simulink model "PID_example_incorrect"  (R2012b)
settings: Solver=ode1  StartTime=0.0  StopTime=80  FixedStep=0.01  RelTol=1e-3
StopFcn:
  | plot(time,[Input simout simout1]);legend('Input','Anti Windup','Incorrect');grid;
  | title('What happens with incorrect implementation')
  | xlabel('Time (sec)');ylabel('Magnitude')
  | shg
undefined symbols (not defined in the file): sigbuilder_block
libraries: simulink x2
settings Model: Creator=JYOGANAN  LastModifiedBy=JYOGANAN

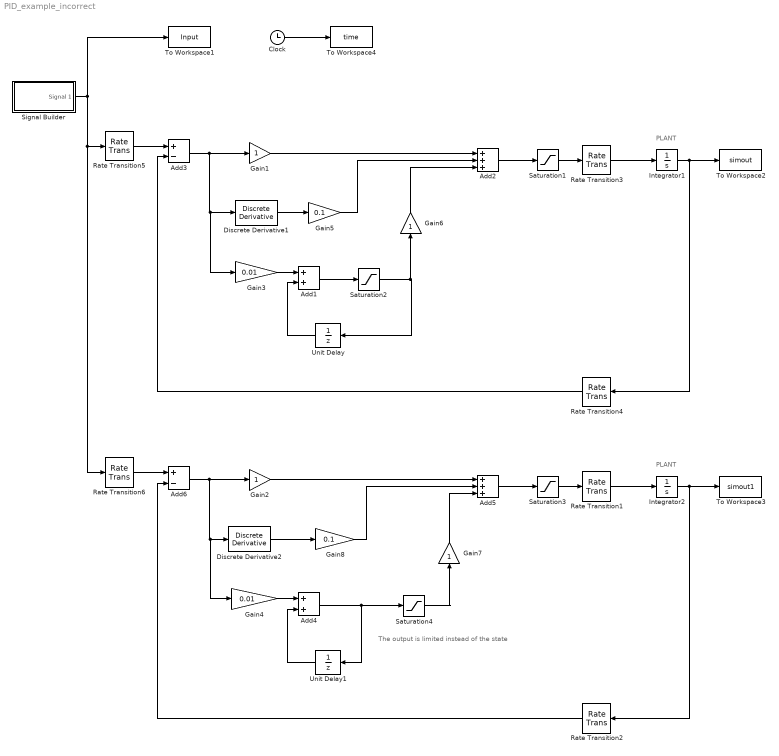
== system PID_example_incorrect ==
  note: The output is limited instead of the state
  note: PLANT
  note: PLANT
  Add1 : Sum
  Add2 : Sum  Inputs=+++
  Add3 : Sum  Inputs=+-
  Add4 : Sum
  Add5 : Sum  Inputs=+++
  Add6 : Sum  Inputs=+-
  Clock : Clock
  Discrete Derivative1 : simulink/Discrete/Discrete Derivative  gainval=1.0  ICPrevScaledInput=0.0  InputProcessing=Inherited  OutMin=[]  OutMax=[]  OutDataType=fixdt(1, 16)  OutScaling=2^-10  DoSatur=off
  Discrete Derivative2 : simulink/Discrete/Discrete Derivative  gainval=1.0  ICPrevScaledInput=0.0  InputProcessing=Inherited  OutMin=[]  OutMax=[]  OutDataType=fixdt(1, 16)  OutScaling=2^-10  DoSatur=off
  Gain{1..2,6..7} (4 alike) : Gain
  Gain3 : Gain  Gain=0.01
  Gain4 : Gain  Gain=0.01
  Gain5 : Gain  Gain=0.1
  Gain8 : Gain  Gain=0.1
  Integrator1 : Integrator
  Integrator2 : Integrator
  Rate Transition1 : RateTransition
  Rate Transition{2,4..6} (4 alike) : RateTransition  OutPortSampleTime=0.01
  Rate Transition3 : RateTransition
  Saturation1 : Saturate  UpperLimit=1  LowerLimit=-1
  Saturation2 : Saturate
  Saturation3 : Saturate  UpperLimit=1  LowerLimit=-1
  Saturation4 : Saturate
  Signal Builder : Subsystem  Tag=STV Subsys  LoadFcn=sigbuilder_block('load');  StartFcn=sigbuilder_block('start');  StopFcn=sigbuilder_block('stop');  ClipboardFcn=sigbuilder_block('clipboard');  mask(Sigbuilder block){}
      mask help: Simulink:masks:SigbuilderBlock_MD
      mask init:
      | if ~strcmp(get_param(bdroot(gcbh),'SimulationStatus'),'stopped') tuvar = sigbuilder_block('maskInit'); end
      settings: CopyFcn=sigbuilder_block('copy');  DeleteFcn=sigbuilder_block('delete');  ModelCloseFcn=sigbuilder_block('modelClose');  PreSaveFcn=sigbuilder_block('preSave');  PauseFcn=sigbuilder_block('pause');  ContinueFcn=sigbuilder_block('continue');  NameChangeFcn=sigbuilder_block('namechange');  OpenFcn=sigbuilder_block('open',[406.5 147 550.5 399.75 ]);  CloseFcn=sigbuilder_block('close');
      mask Display: plot(0, 0, 100, 100,[2, 2, 32, 32, 2], [68, 8, 8, 68, 68],[32, 2], [38, 38], [32, 19, 2],[53, 60, 44], [32, 17, 17, 2],[16, 16, 31, 31]);txt = getActiveGroup(gcbh);text(2, 100, txt,'verticalAlignment', 'top');
  To Workspace1 : ToWorkspace  VariableName=Input  SampleTime=-1
  To Workspace2 : ToWorkspace  VariableName=simout  SampleTime=-1
  To Workspace3 : ToWorkspace  VariableName=simout1  SampleTime=-1
  To Workspace4 : ToWorkspace  VariableName=time  SampleTime=-1
  Unit Delay : UnitDelay  SampleTime=-1
  Unit Delay1 : UnitDelay  SampleTime=-1
  wires:
  Rate Transition3/1 -> Integrator1/1
  Gain1/1 -> Add2/1
  Rate Transition4/1 -> Add3/2
  Integrator1/1 -> To Workspace2/1, Rate Transition4/1
  Rate Transition5/1 -> Add3/1
  Discrete Derivative1/1 -> Gain5/1
  Saturation1/1 -> Rate Transition3/1
  Add2/1 -> Saturation1/1
  Add3/1 -> Gain3/1, Discrete Derivative1/1, Gain1/1
  Signal Builder/1(Signal 1) -> To Workspace1/1, Rate Transition5/1, Rate Transition6/1
  Clock/1 -> To Workspace4/1
  Add1/1 -> Saturation2/1
  Gain3/1 -> Add1/1
  Unit Delay/1 -> Add1/2
  Saturation2/1 -> Unit Delay/1, Gain6/1
  Rate Transition1/1 -> Integrator2/1
  Gain2/1 -> Add5/1
  Rate Transition2/1 -> Add6/2
  Integrator2/1 -> To Workspace3/1, Rate Transition2/1
  Rate Transition6/1 -> Add6/1
  Discrete Derivative2/1 -> Gain8/1
  Saturation3/1 -> Rate Transition1/1
  Add5/1 -> Saturation3/1
  Add6/1 -> Gain4/1, Discrete Derivative2/1, Gain2/1
  Gain4/1 -> Add4/1
  Unit Delay1/1 -> Add4/2
  Add4/1 -> Saturation4/1, Unit Delay1/1
  Saturation4/1 -> Gain7/1
  Gain5/1 -> Add2/2
  Gain6/1 -> Add2/3
  Gain7/1 -> Add5/3
  Gain8/1 -> Add5/2

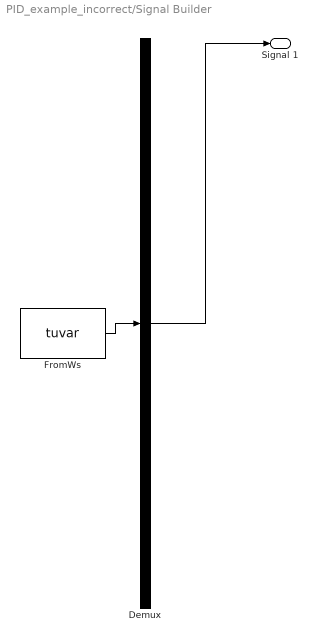
== system PID_example_incorrect/Signal Builder ==
  Demux : Demux  Tag=STV Demux  Outputs=1
  FromWs : FromWorkspace  Tag=STV FromWs  VariableName=tuvar  SampleTime=0
      SigBuilderData=|
      | common.afterFinalStr = 'Extrapolate'
      | common.sampleTime = 0
      | dataSet.timeRange = [0 80]
      | dataSet.name = 'Group 1'
      | sbobj.Groups.Name = 'Group 1'
      | sbobj.Groups.Signals.Name = 'Signal 1'
      | sbobj.Groups.Signals.XData = [0 4.4 4.4 26.2 26.2 60 60 72 72 80]
      | sbobj.Groups.Signals.YData = [0 0 1 1 -1 -1 1 1 0 0]
      | sbobj.Groups.TimeRange = [0 80]
  Signal 1 : Outport  Tag=STV Outport
  wires:
  Demux/1 -> Signal 1/1
  FromWs/1 -> Demux/1
